simulink model "Nils_Modell"  (R2021b)
settings: Solver=FixedStepAuto  StartTime=0.0  StopTime=1  FixedStep=0.001  RelTol=1e-3
values from neighbouring files (symbols this model uses):
  c = 50    [Nils_mfile.m]
  d = 0.05    [Nils_mfile.m]
  dL = 5e-6    (= 5e-06)    [Nils_mfile.m]
  dM = 1.0e-5    (= 1e-05)    [Nils_mfile.m]
  JL = 2e-5    (= 2e-05)    [Nils_mfile.m]
  Jm = 0.125e-5    (= 1.25e-06)    [Nils_mfile.m]
  LM = 1e-3    (= 0.001)    [Nils_mfile.m]
  ML = 0.25    [Nils_mfile.m]
  Oi = 2.6e-2    (= 0.026)    [Nils_mfile.m]
  OM = 0.1125    [Nils_mfile.m]
  rL = 50.0/1000    (= 0.05)    [Nils_mfile.m]
  RM = 1.5    [Nils_mfile.m]
  rM = 25/1000    (= 0.025)    [Nils_mfile.m]
  Uq0 = 24    [Nils_mfile.m]
settings Model: Creator=nilsb  LastModifiedBy=nilsb

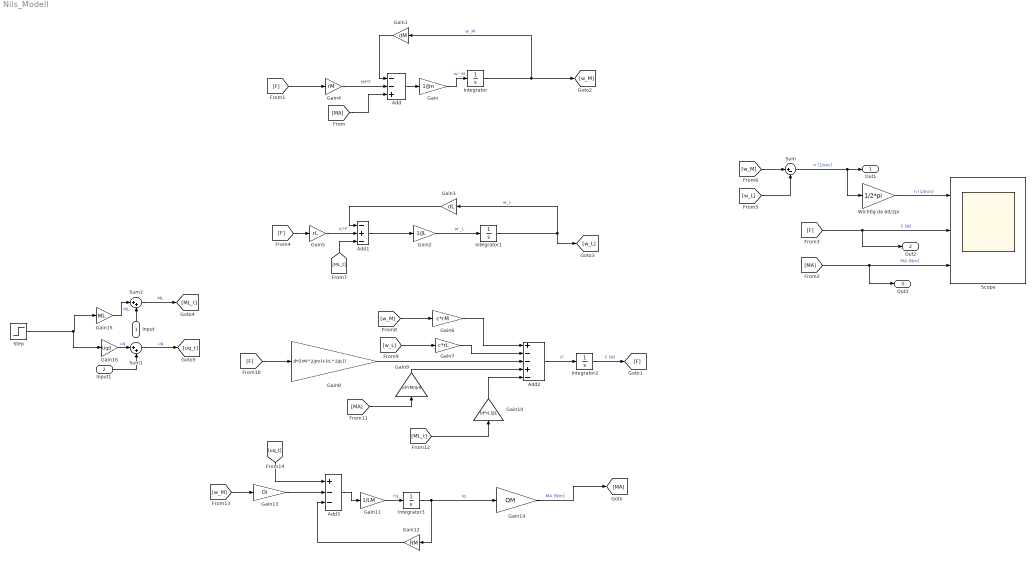
== system Nils_Modell ==
  Input : Inport
  Input1 : Inport  Port=2
  Add : Sum  Inputs=--+
  Add1 : Sum  Inputs=-+-
  Add2 : Sum  Inputs=+--+-
  Add3 : Sum  Inputs=+--
  Gain : Gain  Gain=1/Jm
  Gain1 : Gain  Gain=dM
  Gain10 : Gain  Gain=(d*rL)/JL
  Gain11 : Gain  Gain=1/LM
  Gain12 : Gain  Gain=RM
  Gain13 : Gain  Gain=Oi
  Gain14 : Gain  Gain=OM
  Gain15 : Gain  Gain=ML
  Gain16 : Gain  Gain=Uq0
  Gain2 : Gain  Gain=1/JL
  Gain3 : Gain  Gain=dL
  Gain4 : Gain  Gain=rM
  Gain5 : Gain  Gain=rL
  Gain6 : Gain  Gain=c*rM
  Gain7 : Gain  Gain=c*rL
  Gain8 : Gain  Gain=d*((rM^2/Jm)+(rL^2/JL))
  Gain9 : Gain  Gain=(d*rM)/Jm
  Integrator{,1..3} (4 alike) : Integrator
  Scope : Scope  NumInputPorts=3
  Step : Step  Time=0.1  SampleTime=0
  Sum : Sum  Inputs=|+-
  Sum1 : Sum  Inputs=|++
  Sum2 : Sum  Inputs=|++
  Wichtig da 60/2pi : Gain  Gain=1/2*pi
  Out1 : Outport
  Out2 : Outport  Port=2
  Out3 : Outport  Port=3
  wires:
  Add3/1 -> Gain11/1
  Integrator3/1 -> Gain12/1, Gain14/1  "iq"
  Wichtig da 60/2pi/1 -> Scope/1  "n (1/min)"
  Gain13/1 -> Add3/2
  Gain15/1 -> Sum2/1  "ML"
  Input/1 -> Sum2/2
  Step/1 -> Gain16/1, Gain15/1
  Gain16/1 -> Sum1/1  "uq"
  Input1/1 -> Sum1/2
  Gain6/1 -> Add2/1
  Gain12/1 -> Add3/3
  Gain8/1 -> Add2/3
  Gain9/1 -> Add2/4
  Gain11/1 -> Integrator3/1  "i'q"
  Gain4/1 -> Add/2  "rM*F"
  Sum/1 -> Wichtig da 60/2pi/1, Out1/1  "n (1/sec)"
  Add2/1 -> Integrator2/1  "F'"
  Gain10/1 -> Add2/5
  Gain7/1 -> Add2/2
  Gain3/1 -> Add1/1
  Integrator2/1 -> [F]  "F (N)"
  Add1/1 -> Gain2/1
  Integrator/1 -> [w_M], Gain1/1  "w_M"
  Gain5/1 -> Add1/2  "rL*F"
  Gain14/1 -> [MA]  "MA (Nm)"
  Add/1 -> Gain/1
  Gain1/1 -> Add/1
  Gain2/1 -> Integrator1/1  "w'_L"
  Gain/1 -> Integrator/1  "w'_M"
  Integrator1/1 -> [w_L], Gain3/1  "w_L"
  [MA] -> Add/3
  [F] -> Gain4/1
  [MA] -> Out3/1, Scope/3  "MA (Nm)"
  [F] -> Out2/1, Scope/2  "F (N)"
  [F] -> Gain5/1
  [w_L] -> Sum/2
  [w_M] -> Sum/1
  Sum2/1 -> [ML_t]  "ML"
  Sum1/1 -> [uq_t]  "uq"
  [ML_t] -> Add1/3
  [w_M] -> Gain6/1
  [w_L] -> Gain7/1
  [F] -> Gain8/1
  [MA] -> Gain9/1
  [ML_t] -> Gain10/1
  [w_M] -> Gain13/1
  [uq_t] -> Add3/1
